simulink model "case2"  (R2022b)
settings: Solver=VariableStepAuto  StartTime=0.0  StopTime=30.0  RelTol=1e-3
values from neighbouring files (symbols this model uses):
  Kd_new2 = 0.07    [main.m]
  Ke_new2 = 1.45    [main.m]
undefined symbols (not defined in the file or in its folder): K1_new2, sigbuilder_block
libraries: fuzblock x1
settings Model: Creator=karam  LastModifiedBy=kmpouzio
settings SolverCC: AlgebraicLoopSolver=TrustRegion
settings DebuggingCC: UnconnectedInputMsg=warning  UnconnectedOutputMsg=warning  UnconnectedLineMsg=warning  SFMachineParentedDataDiag=warning
settings ModelReferenceCC: EnableRefExpFcnMdlSchedulingChecks=on

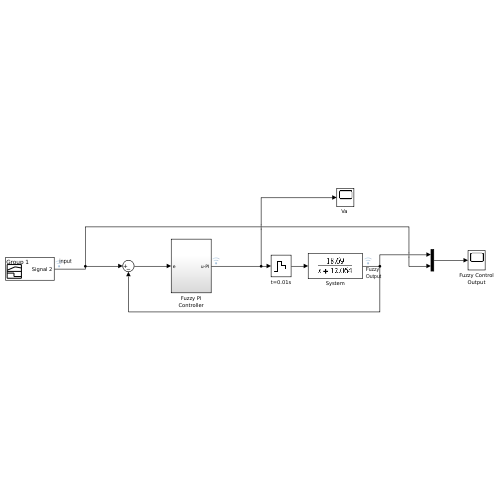
[thumbnail: Simulink's stored preview of the top-level diagram]
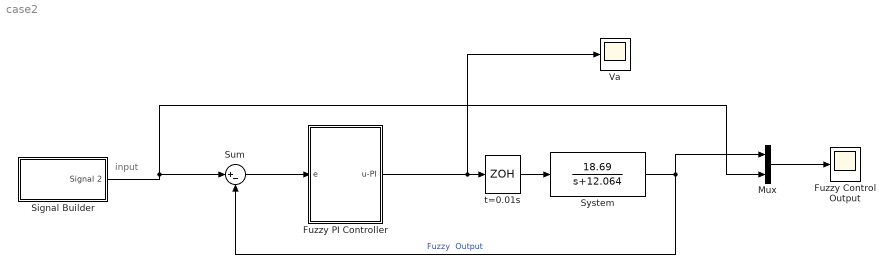
== system case2 ==
  note: input
  Fuzzy Control Output : Scope
  Fuzzy PI Controller : Subsystem
  Mux : Mux  Inputs=2
  Signal Builder : Subsystem  Tag=STV Subsys  LoadFcn=sigbuilder_block('load');  StartFcn=sigbuilder_block('start');  StopFcn=sigbuilder_block('stop');  ClipboardFcn=sigbuilder_block('clipboard');  mask(Sigbuilder block){tuvar=[0:10]}
      mask help: Simulink:masks:SigbuilderBlock_MD
      mask init:
      | if ~strcmp(get_param(bdroot(gcbh),'SimulationStatus'),'stopped') tuvar = sigbuilder_block('maskInit'); end
      settings: CopyFcn=sigbuilder_block('copy');  DeleteFcn=sigbuilder_block('delete');  ModelCloseFcn=sigbuilder_block('modelClose');  PreSaveFcn=sigbuilder_block('preSave');  PauseFcn=sigbuilder_block('pause');  ContinueFcn=sigbuilder_block('continue');  NameChangeFcn=sigbuilder_block('namechange');  OpenFcn=sigbuilder_block('open',[358.2 51 550.8 400.2 ]);  CloseFcn=sigbuilder_block('close');
      mask Display: plot(0, 0, 100, 100,[2, 2, 32, 32, 2], [68, 8, 8, 68, 68],[32, 2], [38, 38], [32, 19, 2],[53, 60, 44], [32, 17, 17, 2],[16, 16, 31, 31]);txt = getActiveGroup(gcbh);text(2, 100, txt,'verticalAlignment', 'top');
  Sum : Sum  Inputs=|+-  SaturateOnIntegerOverflow=on
  System : TransferFcn  Numerator=[18.69]  Denominator=[1 12.064]
  "Va " : Scope
  t=0.01s : ZeroOrderHold  SampleTime=0.01
  wires:
  System/1 -> Sum/2, Mux/1  "Fuzzy  Output"
  Sum/1 -> Fuzzy PI Controller/1(e)
  Mux/1 -> Fuzzy Control Output/1
  Fuzzy PI Controller/1(u-PI) -> "Va "/1, t=0.01s/1
  t=0.01s/1 -> System/1
  Signal Builder/1(Signal 2) -> Sum/1, Mux/2

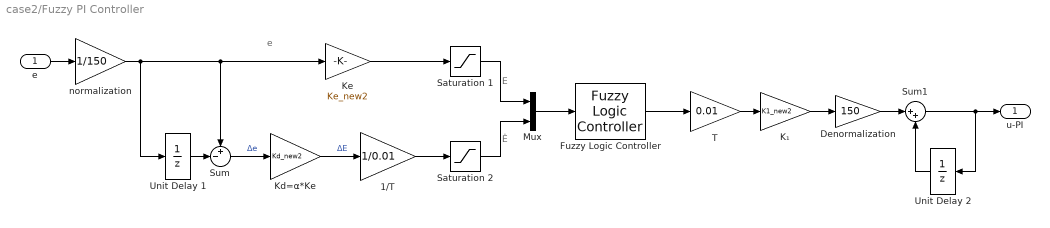
== system case2/Fuzzy PI Controller ==
  note: e
  note: E
  note: Ė
  e : Inport
  1/T : Gain  Gain=1/0.01  SaturateOnIntegerOverflow=on  OutDataTypeStr=Inherit: Same as input  ParamDataTypeStr=Inherit: Same as input
  Denormalization : Gain  Gain=150  SaturateOnIntegerOverflow=on  OutDataTypeStr=Inherit: Same as input  ParamDataTypeStr=Inherit: Same as input
  Fuzzy Logic Controller : fuzblock/Fuzzy Logic  Controller  FIS='FLC07.fis'  OutputSampleNumber=101  DataType=double  FuzzifiedInputs=off  RuleFiringStrengths=off  RuleOutputs=off  AggregatedOutputs=off  SimulateUsing=Interpreted execution  OutOfRangeInputValueMessage=warning  NoRuleFiredMessage=warning  EmptyOutputFuzzySetMessage=warning
  Kd=α*Ke : Gain  Gain=Kd_new2  SaturateOnIntegerOverflow=on  OutDataTypeStr=Inherit: Same as input  ParamDataTypeStr=Inherit: Same as input
  Ke : Gain  Gain=Ke_new2  SaturateOnIntegerOverflow=on  OutDataTypeStr=Inherit: Same as input  ParamDataTypeStr=Inherit: Same as input
  K₁ : Gain  Gain=K1_new2  SaturateOnIntegerOverflow=on  OutDataTypeStr=Inherit: Same as input  ParamDataTypeStr=Inherit: Same as input
  Mux : Mux  Inputs=2
  Saturation 1 : Saturate  UpperLimit=1  LowerLimit=-1
  Saturation 2 : Saturate  UpperLimit=1  LowerLimit=-1
  Sum : Sum  Inputs=+-|  SaturateOnIntegerOverflow=on
  Sum1 : Sum  Inputs=|++  SaturateOnIntegerOverflow=on
  T : Gain  Gain=0.01  SaturateOnIntegerOverflow=on  OutDataTypeStr=Inherit: Same as input  ParamDataTypeStr=Inherit: Same as input
  Unit Delay 1 : UnitDelay  SampleTime=0.01  HasFrameUpgradeWarning=on
  Unit Delay 2 : UnitDelay  SampleTime=0.01  HasFrameUpgradeWarning=on
  normalization : Gain  Gain=1/150  SaturateOnIntegerOverflow=on  OutDataTypeStr=Inherit: Same as input  ParamDataTypeStr=Inherit: Same as input
  u-PI : Outport  VectorParamsAs1DForOutWhenUnconnected=off
  wires:
  e/1 -> normalization/1
  normalization/1 -> Unit Delay 1/1, Ke/1, Sum/1
  Ke/1 -> Saturation 1/1
  Saturation 1/1 -> Mux/1
  T/1 -> K₁/1
  K₁/1 -> Denormalization/1
  Denormalization/1 -> Sum1/1
  Sum1/1 -> u-PI/1, Unit Delay 2/1
  Unit Delay 2/1 -> Sum1/2
  Unit Delay 1/1 -> Sum/2
  Sum/1 -> Kd=α*Ke/1  "Δe"
  Kd=α*Ke/1 -> 1/T/1  "ΔE"
  1/T/1 -> Saturation 2/1
  Saturation 2/1 -> Mux/2
  Mux/1 -> Fuzzy Logic Controller/1
  Fuzzy Logic Controller/1 -> T/1

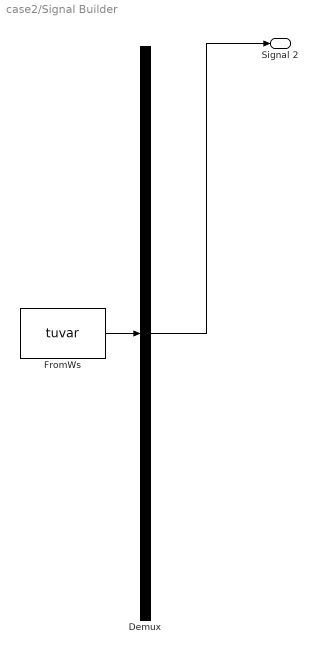
== system case2/Signal Builder ==
  Demux : Demux  Tag=STV Demux  Outputs=1
      settings: DisplayOption=none
  FromWs : FromWorkspace  Tag=STV FromWs  VariableName=tuvar
      SigBuilderData=|
      | common.afterFinalStr = 'Extrapolate'
      | common.sampleTime = '0'
      | dataSet.timeRange = [0 30]
      | dataSet.name = 'Group 1'
      | sbobj.Groups.Name = 'Group 1'
      | sbobj.Groups.Signals.Name = 'Signal 2'
      | sbobj.Groups.Signals.XData = [0 10 20 30]
      | sbobj.Groups.Signals.YData = [0 150 150 0]
      | sbobj.Groups.TimeRange = [0 30]
  Signal 2 : Outport  Tag=STV Outport
  wires:
  FromWs/1 -> Demux/1
  Demux/1 -> Signal 2/1
